simulink model "qr_array"  (R2017a)
settings: Solver=VariableStepAuto  StartTime=0.0  StopTime=777  RelTol=1e-3
libraries: xbsIndex_r4 x646
(part 2 of 4)

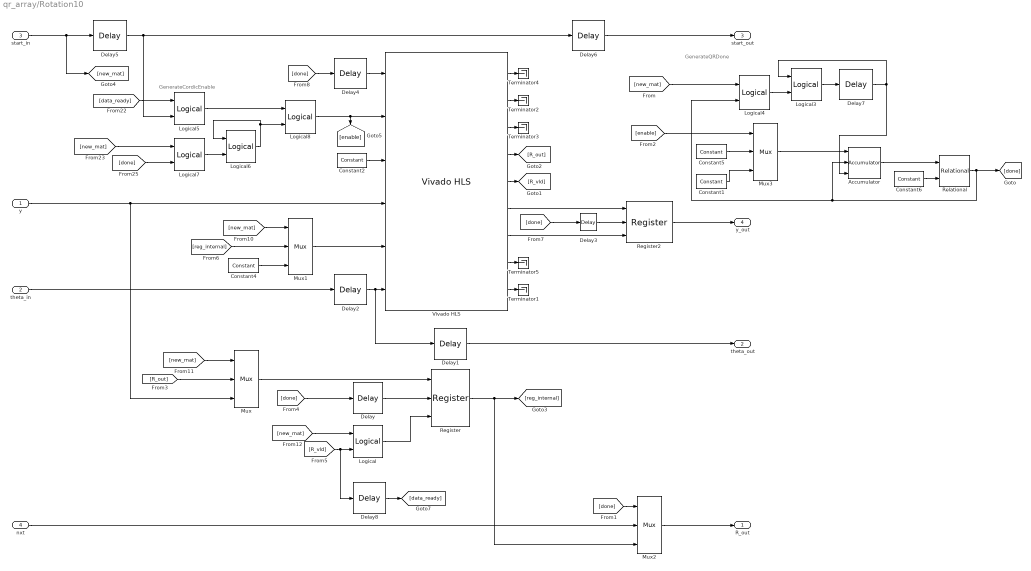
== system qr_array/Rotation10 ==
  note: GenerateQRDone
  note: GenerateCordicEnable
  y : Inport
  theta_in : Inport  Port=2
  start_in : Inport  Port=3
  nxt : Inport  Port=4
  Accumulator : xbsIndex_r4/Accumulator  operation=Add  n_bits=8  overflow=Wrap  scale=1  rst=on  hasbypass=off  infoeditControl=reset for floating point data type must be asserted for a minimum of 2 cycles  en=on  latency=1  msb_inp=100  msb=100  lsb=-100  use_behavioral_HDL=on  implementation=Fabric  dbl_ovrd=off  block_type=accum
  Constant1 : xbsIndex_r4/Constant  const=1  gui_display_data_type=Fixed-point  arith_type=Unsigned  n_bits=16  bin_pt=0  preci_type=Single  exp_width=8  frac_width=24  explicit_period=off  period=1  equ=P=C  opselect=C  inp2=PCIN>>17  opr=+  inp1=P  carry=CIN  dbl_ovrd=off  block_type=constant
  Constant2 : xbsIndex_r4/Constant  const=1  gui_display_data_type=Boolean  arith_type=Boolean  n_bits=16  bin_pt=14  preci_type=Single  exp_width=8  frac_width=24  explicit_period=off  period=1  equ=P=C  opselect=C  inp2=PCIN>>17  opr=+  inp1=P  carry=CIN  dbl_ovrd=off  block_type=constant
  Constant4 : xbsIndex_r4/Constant  const=0  gui_display_data_type=Fixed-point  arith_type=Signed (2's comp)  n_bits=16  bin_pt=13  preci_type=Single  exp_width=8  frac_width=24  explicit_period=off  period=1  equ=P=C  opselect=C  inp2=PCIN>>17  opr=+  inp1=P  carry=CIN  dbl_ovrd=off  block_type=constant
  Constant5 : xbsIndex_r4/Constant  const=0  gui_display_data_type=Fixed-point  arith_type=Unsigned  n_bits=16  bin_pt=0  preci_type=Single  exp_width=8  frac_width=24  explicit_period=off  period=1  equ=P=C  opselect=C  inp2=PCIN>>17  opr=+  inp1=P  carry=CIN  dbl_ovrd=off  block_type=constant
  Constant6 : xbsIndex_r4/Constant  const=3  gui_display_data_type=Fixed-point  arith_type=Unsigned  n_bits=16  bin_pt=0  preci_type=Single  exp_width=8  frac_width=24  explicit_period=off  period=1  equ=P=C  opselect=C  inp2=PCIN>>17  opr=+  inp1=P  carry=CIN  dbl_ovrd=off  block_type=constant
  Delay{,3,6..7} (4 alike) : xbsIndex_r4/Delay  rst=off  infoeditControl=Selection of Reset will increase slice count due to use of real FFs and instead of SRLs  en=off  latency=1  reg_retiming=off  dbl_ovrd=off  block_type=delay
  Delay1 : xbsIndex_r4/Delay  rst=off  infoeditControl=Selection of Reset will increase slice count due to use of real FFs and instead of SRLs  en=off  latency=41  reg_retiming=off  dbl_ovrd=off  block_type=delay
  Delay2 : xbsIndex_r4/Delay  rst=off  infoeditControl=Selection of Reset will increase slice count due to use of real FFs and instead of SRLs  en=off  latency=2  reg_retiming=off  dbl_ovrd=off  block_type=delay
  Delay4 : xbsIndex_r4/Delay  rst=off  infoeditControl=Selection of Reset will increase slice count due to use of real FFs and instead of SRLs  en=off  latency=4  reg_retiming=off  dbl_ovrd=off  block_type=delay
  Delay5 : xbsIndex_r4/Delay  rst=off  infoeditControl=Selection of Reset will increase slice count due to use of real FFs and instead of SRLs  en=off  latency=43  reg_retiming=off  dbl_ovrd=off  block_type=delay
  Delay8 : xbsIndex_r4/Delay  rst=off  infoeditControl=Selection of Reset will increase slice count due to use of real FFs and instead of SRLs  en=off  latency=2  reg_retiming=off  dbl_ovrd=off  block_type=delay
  Logical : xbsIndex_r4/Logical  logical_function=OR  inputs=2  en=off  latency=1  precision=Full  arith_type=Unsigned  n_bits=16  bin_pt=0  align_bp=on  dbl_ovrd=off  block_type=logical
  Logical3 : xbsIndex_r4/Logical  logical_function=XOR  inputs=2  en=off  latency=0  precision=Full  arith_type=Unsigned  n_bits=16  bin_pt=0  align_bp=on  dbl_ovrd=off  block_type=logical
  Logical4 : xbsIndex_r4/Logical  logical_function=OR  inputs=2  en=off  latency=1  precision=Full  arith_type=Unsigned  n_bits=16  bin_pt=0  align_bp=on  dbl_ovrd=off  block_type=logical
  Logical5 : xbsIndex_r4/Logical  logical_function=OR  inputs=2  en=off  latency=0  precision=Full  arith_type=Unsigned  n_bits=16  bin_pt=0  align_bp=on  dbl_ovrd=off  block_type=logical
  Logical6 : xbsIndex_r4/Logical  logical_function=XOR  inputs=2  en=off  latency=1  precision=Full  arith_type=Unsigned  n_bits=16  bin_pt=0  align_bp=on  dbl_ovrd=off  block_type=logical
  Logical7 : xbsIndex_r4/Logical  logical_function=OR  inputs=2  en=off  latency=1  precision=Full  arith_type=Unsigned  n_bits=16  bin_pt=0  align_bp=on  dbl_ovrd=off  block_type=logical
  Logical8 : xbsIndex_r4/Logical  logical_function=AND  inputs=2  en=off  latency=1  precision=Full  arith_type=Unsigned  n_bits=16  bin_pt=0  align_bp=on  dbl_ovrd=off  block_type=logical
  Mux{,1..3} (4 alike) : xbsIndex_r4/Mux  inputs=2  en=off  latency=1  precision=Full  arith_type=Unsigned  n_bits=16  bin_pt=14  quantization=Truncate  overflow=Wrap  dbl_ovrd=off  block_type=mux
  Register : xbsIndex_r4/Register  init=0  rst=on  en=on  dbl_ovrd=off  block_type=register
  Register2 : xbsIndex_r4/Register  init=0  rst=on  en=on  dbl_ovrd=off  block_type=register
  Relational : xbsIndex_r4/Relational  mode=a=b  op_type=Bool  en=off  latency=0  dbl_ovrd=off  block_type=relational
  Terminator{1..5} (5 alike) : Terminator
  Vivado HLS : xbsIndex_r4/Vivado HLS  anytable='C:/ELEC522/hellar/Project_4/cordic_revised/cordic_revised/solution1'  fast_sim=off  display_datatype=on  rate_propagation_method=Simulink system period  model_file_path=''  latency=1  block_type=hls
      settings: infoedit=This block allows including C,C++ and SystemC source files in System Generator for DSP designs.
  R_out : Outport
  theta_out : Outport  Port=2
  start_out : Outport  Port=3
  y_out : Outport  Port=4
  wires:
  [done] -> Delay3/1
  Delay8/1 -> [data_ready]
  [R_vld] -> Delay8/1, Logical/2
  [done] -> Mux2/1
  [new_mat] -> Mux/1
  [done] -> Delay4/1
  [new_mat] -> Mux1/1
  [reg_internal] -> Mux1/2
  Delay4/1 -> Vivado HLS/1
  Logical/1 -> Register/3
  [done] -> Delay/1
  [new_mat] -> Logical/1
  theta_in/1 -> Delay2/1
  Register/1 -> Mux2/3, [reg_internal]
  Delay6/1 -> start_out/1
  Mux/1 -> Register/1
  Vivado HLS/3 -> Terminator3/1
  Vivado HLS/5 -> [R_vld]
  [R_out] -> Mux/2
  Delay/1 -> Register/2
  y/1 -> Vivado HLS/4, Mux/3
  Vivado HLS/1 -> Terminator4/1
  Vivado HLS/4 -> [R_out]
  Mux2/1 -> R_out/1
  Constant4/1 -> Mux1/3
  start_in/1 -> [new_mat], Delay5/1
  nxt/1 -> Mux2/2
  Vivado HLS/2 -> Terminator2/1
  Constant2/1 -> Vivado HLS/3
  Logical8/1 -> Vivado HLS/2, [enable]
  Relational/1 -> Logical4/2, Accumulator/2, [done]
  Vivado HLS/8 -> Terminator5/1
  Vivado HLS/9 -> Terminator1/1
  Vivado HLS/6 -> Register2/1
  Vivado HLS/7 -> Register2/3
  Delay1/1 -> theta_out/1
  Delay2/1 -> Delay1/1, Vivado HLS/6
  Mux1/1 -> Vivado HLS/5
  Delay3/1 -> Register2/2
  Register2/1 -> y_out/1
  Logical5/1 -> Logical8/1
  Logical7/1 -> Logical6/2
  Logical6/1 -> Logical6/1, Logical8/2
  [done] -> Logical7/2
  [new_mat] -> Logical7/1
  [data_ready] -> Logical5/1
  Delay5/1 -> Delay6/1, Logical5/2
  Delay7/1 -> Logical3/1, Accumulator/3
  Logical3/1 -> Delay7/1
  Logical4/1 -> Logical3/2
  [new_mat] -> Logical4/1
  Constant6/1 -> Relational/2
  Constant5/1 -> Mux3/2
  Constant1/1 -> Mux3/3
  Accumulator/1 -> Relational/1
  Mux3/1 -> Accumulator/1
  [enable] -> Mux3/1

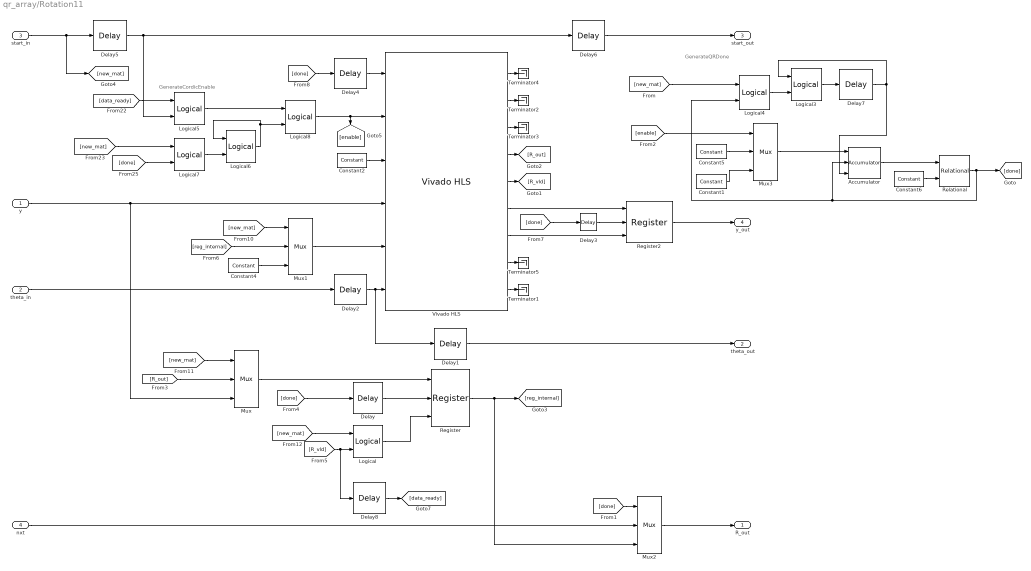
== system qr_array/Rotation11 ==
  note: GenerateQRDone
  note: GenerateCordicEnable
  y : Inport
  theta_in : Inport  Port=2
  start_in : Inport  Port=3
  nxt : Inport  Port=4
  Accumulator : xbsIndex_r4/Accumulator  operation=Add  n_bits=8  overflow=Wrap  scale=1  rst=on  hasbypass=off  infoeditControl=reset for floating point data type must be asserted for a minimum of 2 cycles  en=on  latency=1  msb_inp=100  msb=100  lsb=-100  use_behavioral_HDL=on  implementation=Fabric  dbl_ovrd=off  block_type=accum
  Constant1 : xbsIndex_r4/Constant  const=1  gui_display_data_type=Fixed-point  arith_type=Unsigned  n_bits=16  bin_pt=0  preci_type=Single  exp_width=8  frac_width=24  explicit_period=off  period=1  equ=P=C  opselect=C  inp2=PCIN>>17  opr=+  inp1=P  carry=CIN  dbl_ovrd=off  block_type=constant
  Constant2 : xbsIndex_r4/Constant  const=1  gui_display_data_type=Boolean  arith_type=Boolean  n_bits=16  bin_pt=14  preci_type=Single  exp_width=8  frac_width=24  explicit_period=off  period=1  equ=P=C  opselect=C  inp2=PCIN>>17  opr=+  inp1=P  carry=CIN  dbl_ovrd=off  block_type=constant
  Constant4 : xbsIndex_r4/Constant  const=0  gui_display_data_type=Fixed-point  arith_type=Signed (2's comp)  n_bits=16  bin_pt=13  preci_type=Single  exp_width=8  frac_width=24  explicit_period=off  period=1  equ=P=C  opselect=C  inp2=PCIN>>17  opr=+  inp1=P  carry=CIN  dbl_ovrd=off  block_type=constant
  Constant5 : xbsIndex_r4/Constant  const=0  gui_display_data_type=Fixed-point  arith_type=Unsigned  n_bits=16  bin_pt=0  preci_type=Single  exp_width=8  frac_width=24  explicit_period=off  period=1  equ=P=C  opselect=C  inp2=PCIN>>17  opr=+  inp1=P  carry=CIN  dbl_ovrd=off  block_type=constant
  Constant6 : xbsIndex_r4/Constant  const=3  gui_display_data_type=Fixed-point  arith_type=Unsigned  n_bits=16  bin_pt=0  preci_type=Single  exp_width=8  frac_width=24  explicit_period=off  period=1  equ=P=C  opselect=C  inp2=PCIN>>17  opr=+  inp1=P  carry=CIN  dbl_ovrd=off  block_type=constant
  Delay{,3,6..7} (4 alike) : xbsIndex_r4/Delay  rst=off  infoeditControl=Selection of Reset will increase slice count due to use of real FFs and instead of SRLs  en=off  latency=1  reg_retiming=off  dbl_ovrd=off  block_type=delay
  Delay1 : xbsIndex_r4/Delay  rst=off  infoeditControl=Selection of Reset will increase slice count due to use of real FFs and instead of SRLs  en=off  latency=41  reg_retiming=off  dbl_ovrd=off  block_type=delay
  Delay2 : xbsIndex_r4/Delay  rst=off  infoeditControl=Selection of Reset will increase slice count due to use of real FFs and instead of SRLs  en=off  latency=2  reg_retiming=off  dbl_ovrd=off  block_type=delay
  Delay4 : xbsIndex_r4/Delay  rst=off  infoeditControl=Selection of Reset will increase slice count due to use of real FFs and instead of SRLs  en=off  latency=4  reg_retiming=off  dbl_ovrd=off  block_type=delay
  Delay5 : xbsIndex_r4/Delay  rst=off  infoeditControl=Selection of Reset will increase slice count due to use of real FFs and instead of SRLs  en=off  latency=43  reg_retiming=off  dbl_ovrd=off  block_type=delay
  Delay8 : xbsIndex_r4/Delay  rst=off  infoeditControl=Selection of Reset will increase slice count due to use of real FFs and instead of SRLs  en=off  latency=2  reg_retiming=off  dbl_ovrd=off  block_type=delay
  Logical : xbsIndex_r4/Logical  logical_function=OR  inputs=2  en=off  latency=1  precision=Full  arith_type=Unsigned  n_bits=16  bin_pt=0  align_bp=on  dbl_ovrd=off  block_type=logical
  Logical3 : xbsIndex_r4/Logical  logical_function=XOR  inputs=2  en=off  latency=0  precision=Full  arith_type=Unsigned  n_bits=16  bin_pt=0  align_bp=on  dbl_ovrd=off  block_type=logical
  Logical4 : xbsIndex_r4/Logical  logical_function=OR  inputs=2  en=off  latency=1  precision=Full  arith_type=Unsigned  n_bits=16  bin_pt=0  align_bp=on  dbl_ovrd=off  block_type=logical
  Logical5 : xbsIndex_r4/Logical  logical_function=OR  inputs=2  en=off  latency=0  precision=Full  arith_type=Unsigned  n_bits=16  bin_pt=0  align_bp=on  dbl_ovrd=off  block_type=logical
  Logical6 : xbsIndex_r4/Logical  logical_function=XOR  inputs=2  en=off  latency=1  precision=Full  arith_type=Unsigned  n_bits=16  bin_pt=0  align_bp=on  dbl_ovrd=off  block_type=logical
  Logical7 : xbsIndex_r4/Logical  logical_function=OR  inputs=2  en=off  latency=1  precision=Full  arith_type=Unsigned  n_bits=16  bin_pt=0  align_bp=on  dbl_ovrd=off  block_type=logical
  Logical8 : xbsIndex_r4/Logical  logical_function=AND  inputs=2  en=off  latency=1  precision=Full  arith_type=Unsigned  n_bits=16  bin_pt=0  align_bp=on  dbl_ovrd=off  block_type=logical
  Mux{,1..3} (4 alike) : xbsIndex_r4/Mux  inputs=2  en=off  latency=1  precision=Full  arith_type=Unsigned  n_bits=16  bin_pt=14  quantization=Truncate  overflow=Wrap  dbl_ovrd=off  block_type=mux
  Register : xbsIndex_r4/Register  init=0  rst=on  en=on  dbl_ovrd=off  block_type=register
  Register2 : xbsIndex_r4/Register  init=0  rst=on  en=on  dbl_ovrd=off  block_type=register
  Relational : xbsIndex_r4/Relational  mode=a=b  op_type=Bool  en=off  latency=0  dbl_ovrd=off  block_type=relational
  Terminator{1..5} (5 alike) : Terminator
  Vivado HLS : xbsIndex_r4/Vivado HLS  anytable='C:/ELEC522/hellar/Project_4/cordic_revised/cordic_revised/solution1'  fast_sim=off  display_datatype=on  rate_propagation_method=Simulink system period  model_file_path=''  latency=1  block_type=hls
      settings: infoedit=This block allows including C,C++ and SystemC source files in System Generator for DSP designs.
  R_out : Outport
  theta_out : Outport  Port=2
  start_out : Outport  Port=3
  y_out : Outport  Port=4
  wires:
  [done] -> Delay3/1
  Delay8/1 -> [data_ready]
  [R_vld] -> Delay8/1, Logical/2
  [done] -> Mux2/1
  [new_mat] -> Mux/1
  [done] -> Delay4/1
  [new_mat] -> Mux1/1
  [reg_internal] -> Mux1/2
  Delay4/1 -> Vivado HLS/1
  Logical/1 -> Register/3
  [done] -> Delay/1
  [new_mat] -> Logical/1
  theta_in/1 -> Delay2/1
  Register/1 -> Mux2/3, [reg_internal]
  Delay6/1 -> start_out/1
  Mux/1 -> Register/1
  Vivado HLS/3 -> Terminator3/1
  Vivado HLS/5 -> [R_vld]
  [R_out] -> Mux/2
  Delay/1 -> Register/2
  y/1 -> Vivado HLS/4, Mux/3
  Vivado HLS/1 -> Terminator4/1
  Vivado HLS/4 -> [R_out]
  Mux2/1 -> R_out/1
  Constant4/1 -> Mux1/3
  start_in/1 -> [new_mat], Delay5/1
  nxt/1 -> Mux2/2
  Vivado HLS/2 -> Terminator2/1
  Constant2/1 -> Vivado HLS/3
  Logical8/1 -> Vivado HLS/2, [enable]
  Relational/1 -> Logical4/2, Accumulator/2, [done]
  Vivado HLS/8 -> Terminator5/1
  Vivado HLS/9 -> Terminator1/1
  Vivado HLS/6 -> Register2/1
  Vivado HLS/7 -> Register2/3
  Delay1/1 -> theta_out/1
  Delay2/1 -> Delay1/1, Vivado HLS/6
  Mux1/1 -> Vivado HLS/5
  Delay3/1 -> Register2/2
  Register2/1 -> y_out/1
  Logical5/1 -> Logical8/1
  Logical7/1 -> Logical6/2
  Logical6/1 -> Logical6/1, Logical8/2
  [done] -> Logical7/2
  [new_mat] -> Logical7/1
  [data_ready] -> Logical5/1
  Delay5/1 -> Delay6/1, Logical5/2
  Delay7/1 -> Logical3/1, Accumulator/3
  Logical3/1 -> Delay7/1
  Logical4/1 -> Logical3/2
  [new_mat] -> Logical4/1
  Constant6/1 -> Relational/2
  Constant5/1 -> Mux3/2
  Constant1/1 -> Mux3/3
  Accumulator/1 -> Relational/1
  Mux3/1 -> Accumulator/1
  [enable] -> Mux3/1

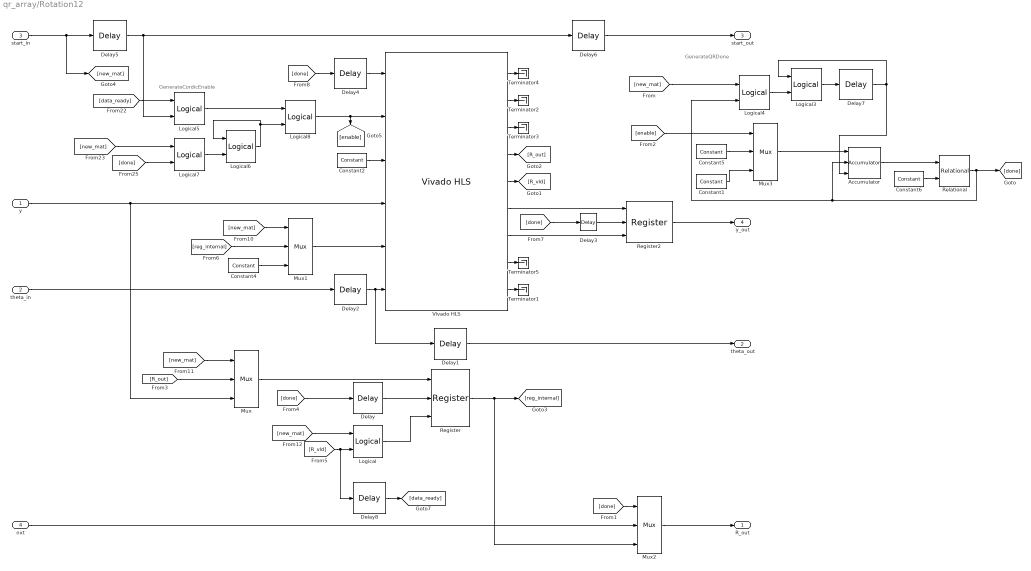
== system qr_array/Rotation12 ==
  note: GenerateQRDone
  note: GenerateCordicEnable
  y : Inport
  theta_in : Inport  Port=2
  start_in : Inport  Port=3
  nxt : Inport  Port=4
  Accumulator : xbsIndex_r4/Accumulator  operation=Add  n_bits=8  overflow=Wrap  scale=1  rst=on  hasbypass=off  infoeditControl=reset for floating point data type must be asserted for a minimum of 2 cycles  en=on  latency=1  msb_inp=100  msb=100  lsb=-100  use_behavioral_HDL=on  implementation=Fabric  dbl_ovrd=off  block_type=accum
  Constant1 : xbsIndex_r4/Constant  const=1  gui_display_data_type=Fixed-point  arith_type=Unsigned  n_bits=16  bin_pt=0  preci_type=Single  exp_width=8  frac_width=24  explicit_period=off  period=1  equ=P=C  opselect=C  inp2=PCIN>>17  opr=+  inp1=P  carry=CIN  dbl_ovrd=off  block_type=constant
  Constant2 : xbsIndex_r4/Constant  const=1  gui_display_data_type=Boolean  arith_type=Boolean  n_bits=16  bin_pt=14  preci_type=Single  exp_width=8  frac_width=24  explicit_period=off  period=1  equ=P=C  opselect=C  inp2=PCIN>>17  opr=+  inp1=P  carry=CIN  dbl_ovrd=off  block_type=constant
  Constant4 : xbsIndex_r4/Constant  const=0  gui_display_data_type=Fixed-point  arith_type=Signed (2's comp)  n_bits=16  bin_pt=13  preci_type=Single  exp_width=8  frac_width=24  explicit_period=off  period=1  equ=P=C  opselect=C  inp2=PCIN>>17  opr=+  inp1=P  carry=CIN  dbl_ovrd=off  block_type=constant
  Constant5 : xbsIndex_r4/Constant  const=0  gui_display_data_type=Fixed-point  arith_type=Unsigned  n_bits=16  bin_pt=0  preci_type=Single  exp_width=8  frac_width=24  explicit_period=off  period=1  equ=P=C  opselect=C  inp2=PCIN>>17  opr=+  inp1=P  carry=CIN  dbl_ovrd=off  block_type=constant
  Constant6 : xbsIndex_r4/Constant  const=2  gui_display_data_type=Fixed-point  arith_type=Unsigned  n_bits=16  bin_pt=0  preci_type=Single  exp_width=8  frac_width=24  explicit_period=off  period=1  equ=P=C  opselect=C  inp2=PCIN>>17  opr=+  inp1=P  carry=CIN  dbl_ovrd=off  block_type=constant
  Delay{,3,6..7} (4 alike) : xbsIndex_r4/Delay  rst=off  infoeditControl=Selection of Reset will increase slice count due to use of real FFs and instead of SRLs  en=off  latency=1  reg_retiming=off  dbl_ovrd=off  block_type=delay
  Delay1 : xbsIndex_r4/Delay  rst=off  infoeditControl=Selection of Reset will increase slice count due to use of real FFs and instead of SRLs  en=off  latency=41  reg_retiming=off  dbl_ovrd=off  block_type=delay
  Delay2 : xbsIndex_r4/Delay  rst=off  infoeditControl=Selection of Reset will increase slice count due to use of real FFs and instead of SRLs  en=off  latency=2  reg_retiming=off  dbl_ovrd=off  block_type=delay
  Delay4 : xbsIndex_r4/Delay  rst=off  infoeditControl=Selection of Reset will increase slice count due to use of real FFs and instead of SRLs  en=off  latency=4  reg_retiming=off  dbl_ovrd=off  block_type=delay
  Delay5 : xbsIndex_r4/Delay  rst=off  infoeditControl=Selection of Reset will increase slice count due to use of real FFs and instead of SRLs  en=off  latency=43  reg_retiming=off  dbl_ovrd=off  block_type=delay
  Delay8 : xbsIndex_r4/Delay  rst=off  infoeditControl=Selection of Reset will increase slice count due to use of real FFs and instead of SRLs  en=off  latency=2  reg_retiming=off  dbl_ovrd=off  block_type=delay
  Logical : xbsIndex_r4/Logical  logical_function=OR  inputs=2  en=off  latency=1  precision=Full  arith_type=Unsigned  n_bits=16  bin_pt=0  align_bp=on  dbl_ovrd=off  block_type=logical
  Logical3 : xbsIndex_r4/Logical  logical_function=XOR  inputs=2  en=off  latency=0  precision=Full  arith_type=Unsigned  n_bits=16  bin_pt=0  align_bp=on  dbl_ovrd=off  block_type=logical
  Logical4 : xbsIndex_r4/Logical  logical_function=OR  inputs=2  en=off  latency=1  precision=Full  arith_type=Unsigned  n_bits=16  bin_pt=0  align_bp=on  dbl_ovrd=off  block_type=logical
  Logical5 : xbsIndex_r4/Logical  logical_function=OR  inputs=2  en=off  latency=0  precision=Full  arith_type=Unsigned  n_bits=16  bin_pt=0  align_bp=on  dbl_ovrd=off  block_type=logical
  Logical6 : xbsIndex_r4/Logical  logical_function=XOR  inputs=2  en=off  latency=1  precision=Full  arith_type=Unsigned  n_bits=16  bin_pt=0  align_bp=on  dbl_ovrd=off  block_type=logical
  Logical7 : xbsIndex_r4/Logical  logical_function=OR  inputs=2  en=off  latency=1  precision=Full  arith_type=Unsigned  n_bits=16  bin_pt=0  align_bp=on  dbl_ovrd=off  block_type=logical
  Logical8 : xbsIndex_r4/Logical  logical_function=AND  inputs=2  en=off  latency=1  precision=Full  arith_type=Unsigned  n_bits=16  bin_pt=0  align_bp=on  dbl_ovrd=off  block_type=logical
  Mux{,1..3} (4 alike) : xbsIndex_r4/Mux  inputs=2  en=off  latency=1  precision=Full  arith_type=Unsigned  n_bits=16  bin_pt=14  quantization=Truncate  overflow=Wrap  dbl_ovrd=off  block_type=mux
  Register : xbsIndex_r4/Register  init=0  rst=on  en=on  dbl_ovrd=off  block_type=register
  Register2 : xbsIndex_r4/Register  init=0  rst=on  en=on  dbl_ovrd=off  block_type=register
  Relational : xbsIndex_r4/Relational  mode=a=b  op_type=Bool  en=off  latency=0  dbl_ovrd=off  block_type=relational
  Terminator{1..5} (5 alike) : Terminator
  Vivado HLS : xbsIndex_r4/Vivado HLS  anytable='C:/ELEC522/hellar/Project_4/cordic_revised/cordic_revised/solution1'  fast_sim=off  display_datatype=on  rate_propagation_method=Simulink system period  model_file_path=''  latency=1  block_type=hls
      settings: infoedit=This block allows including C,C++ and SystemC source files in System Generator for DSP designs.
  R_out : Outport
  theta_out : Outport  Port=2
  start_out : Outport  Port=3
  y_out : Outport  Port=4
  wires:
  [done] -> Delay3/1
  Delay8/1 -> [data_ready]
  [R_vld] -> Delay8/1, Logical/2
  [done] -> Mux2/1
  [new_mat] -> Mux/1
  [done] -> Delay4/1
  [new_mat] -> Mux1/1
  [reg_internal] -> Mux1/2
  Delay4/1 -> Vivado HLS/1
  Logical/1 -> Register/3
  [done] -> Delay/1
  [new_mat] -> Logical/1
  theta_in/1 -> Delay2/1
  Register/1 -> Mux2/3, [reg_internal]
  Delay6/1 -> start_out/1
  Mux/1 -> Register/1
  Vivado HLS/3 -> Terminator3/1
  Vivado HLS/5 -> [R_vld]
  [R_out] -> Mux/2
  Delay/1 -> Register/2
  y/1 -> Vivado HLS/4, Mux/3
  Vivado HLS/1 -> Terminator4/1
  Vivado HLS/4 -> [R_out]
  Mux2/1 -> R_out/1
  Constant4/1 -> Mux1/3
  start_in/1 -> [new_mat], Delay5/1
  nxt/1 -> Mux2/2
  Vivado HLS/2 -> Terminator2/1
  Constant2/1 -> Vivado HLS/3
  Logical8/1 -> Vivado HLS/2, [enable]
  Relational/1 -> Logical4/2, Accumulator/2, [done]
  Vivado HLS/8 -> Terminator5/1
  Vivado HLS/9 -> Terminator1/1
  Vivado HLS/6 -> Register2/1
  Vivado HLS/7 -> Register2/3
  Delay1/1 -> theta_out/1
  Delay2/1 -> Delay1/1, Vivado HLS/6
  Mux1/1 -> Vivado HLS/5
  Delay3/1 -> Register2/2
  Register2/1 -> y_out/1
  Logical5/1 -> Logical8/1
  Logical7/1 -> Logical6/2
  Logical6/1 -> Logical6/1, Logical8/2
  [done] -> Logical7/2
  [new_mat] -> Logical7/1
  [data_ready] -> Logical5/1
  Delay5/1 -> Delay6/1, Logical5/2
  Delay7/1 -> Logical3/1, Accumulator/3
  Logical3/1 -> Delay7/1
  Logical4/1 -> Logical3/2
  [new_mat] -> Logical4/1
  Constant6/1 -> Relational/2
  Constant5/1 -> Mux3/2
  Constant1/1 -> Mux3/3
  Accumulator/1 -> Relational/1
  Mux3/1 -> Accumulator/1
  [enable] -> Mux3/1

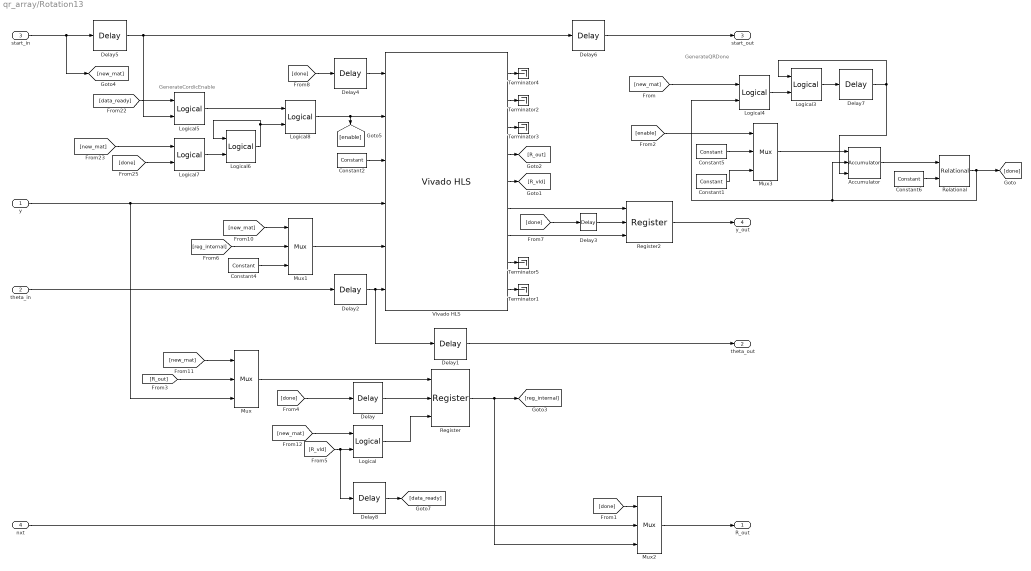
== system qr_array/Rotation13 ==
  note: GenerateQRDone
  note: GenerateCordicEnable
  y : Inport
  theta_in : Inport  Port=2
  start_in : Inport  Port=3
  nxt : Inport  Port=4
  Accumulator : xbsIndex_r4/Accumulator  operation=Add  n_bits=8  overflow=Wrap  scale=1  rst=on  hasbypass=off  infoeditControl=reset for floating point data type must be asserted for a minimum of 2 cycles  en=on  latency=1  msb_inp=100  msb=100  lsb=-100  use_behavioral_HDL=on  implementation=Fabric  dbl_ovrd=off  block_type=accum
  Constant1 : xbsIndex_r4/Constant  const=1  gui_display_data_type=Fixed-point  arith_type=Unsigned  n_bits=16  bin_pt=0  preci_type=Single  exp_width=8  frac_width=24  explicit_period=off  period=1  equ=P=C  opselect=C  inp2=PCIN>>17  opr=+  inp1=P  carry=CIN  dbl_ovrd=off  block_type=constant
  Constant2 : xbsIndex_r4/Constant  const=1  gui_display_data_type=Boolean  arith_type=Boolean  n_bits=16  bin_pt=14  preci_type=Single  exp_width=8  frac_width=24  explicit_period=off  period=1  equ=P=C  opselect=C  inp2=PCIN>>17  opr=+  inp1=P  carry=CIN  dbl_ovrd=off  block_type=constant
  Constant4 : xbsIndex_r4/Constant  const=0  gui_display_data_type=Fixed-point  arith_type=Signed (2's comp)  n_bits=16  bin_pt=13  preci_type=Single  exp_width=8  frac_width=24  explicit_period=off  period=1  equ=P=C  opselect=C  inp2=PCIN>>17  opr=+  inp1=P  carry=CIN  dbl_ovrd=off  block_type=constant
  Constant5 : xbsIndex_r4/Constant  const=0  gui_display_data_type=Fixed-point  arith_type=Unsigned  n_bits=16  bin_pt=0  preci_type=Single  exp_width=8  frac_width=24  explicit_period=off  period=1  equ=P=C  opselect=C  inp2=PCIN>>17  opr=+  inp1=P  carry=CIN  dbl_ovrd=off  block_type=constant
  Constant6 : xbsIndex_r4/Constant  const=2  gui_display_data_type=Fixed-point  arith_type=Unsigned  n_bits=16  bin_pt=0  preci_type=Single  exp_width=8  frac_width=24  explicit_period=off  period=1  equ=P=C  opselect=C  inp2=PCIN>>17  opr=+  inp1=P  carry=CIN  dbl_ovrd=off  block_type=constant
  Delay{,3,6..7} (4 alike) : xbsIndex_r4/Delay  rst=off  infoeditControl=Selection of Reset will increase slice count due to use of real FFs and instead of SRLs  en=off  latency=1  reg_retiming=off  dbl_ovrd=off  block_type=delay
  Delay1 : xbsIndex_r4/Delay  rst=off  infoeditControl=Selection of Reset will increase slice count due to use of real FFs and instead of SRLs  en=off  latency=41  reg_retiming=off  dbl_ovrd=off  block_type=delay
  Delay2 : xbsIndex_r4/Delay  rst=off  infoeditControl=Selection of Reset will increase slice count due to use of real FFs and instead of SRLs  en=off  latency=2  reg_retiming=off  dbl_ovrd=off  block_type=delay
  Delay4 : xbsIndex_r4/Delay  rst=off  infoeditControl=Selection of Reset will increase slice count due to use of real FFs and instead of SRLs  en=off  latency=4  reg_retiming=off  dbl_ovrd=off  block_type=delay
  Delay5 : xbsIndex_r4/Delay  rst=off  infoeditControl=Selection of Reset will increase slice count due to use of real FFs and instead of SRLs  en=off  latency=43  reg_retiming=off  dbl_ovrd=off  block_type=delay
  Delay8 : xbsIndex_r4/Delay  rst=off  infoeditControl=Selection of Reset will increase slice count due to use of real FFs and instead of SRLs  en=off  latency=2  reg_retiming=off  dbl_ovrd=off  block_type=delay
  Logical : xbsIndex_r4/Logical  logical_function=OR  inputs=2  en=off  latency=1  precision=Full  arith_type=Unsigned  n_bits=16  bin_pt=0  align_bp=on  dbl_ovrd=off  block_type=logical
  Logical3 : xbsIndex_r4/Logical  logical_function=XOR  inputs=2  en=off  latency=0  precision=Full  arith_type=Unsigned  n_bits=16  bin_pt=0  align_bp=on  dbl_ovrd=off  block_type=logical
  Logical4 : xbsIndex_r4/Logical  logical_function=OR  inputs=2  en=off  latency=1  precision=Full  arith_type=Unsigned  n_bits=16  bin_pt=0  align_bp=on  dbl_ovrd=off  block_type=logical
  Logical5 : xbsIndex_r4/Logical  logical_function=OR  inputs=2  en=off  latency=0  precision=Full  arith_type=Unsigned  n_bits=16  bin_pt=0  align_bp=on  dbl_ovrd=off  block_type=logical
  Logical6 : xbsIndex_r4/Logical  logical_function=XOR  inputs=2  en=off  latency=1  precision=Full  arith_type=Unsigned  n_bits=16  bin_pt=0  align_bp=on  dbl_ovrd=off  block_type=logical
  Logical7 : xbsIndex_r4/Logical  logical_function=OR  inputs=2  en=off  latency=1  precision=Full  arith_type=Unsigned  n_bits=16  bin_pt=0  align_bp=on  dbl_ovrd=off  block_type=logical
  Logical8 : xbsIndex_r4/Logical  logical_function=AND  inputs=2  en=off  latency=1  precision=Full  arith_type=Unsigned  n_bits=16  bin_pt=0  align_bp=on  dbl_ovrd=off  block_type=logical
  Mux{,1..3} (4 alike) : xbsIndex_r4/Mux  inputs=2  en=off  latency=1  precision=Full  arith_type=Unsigned  n_bits=16  bin_pt=14  quantization=Truncate  overflow=Wrap  dbl_ovrd=off  block_type=mux
  Register : xbsIndex_r4/Register  init=0  rst=on  en=on  dbl_ovrd=off  block_type=register
  Register2 : xbsIndex_r4/Register  init=0  rst=on  en=on  dbl_ovrd=off  block_type=register
  Relational : xbsIndex_r4/Relational  mode=a=b  op_type=Bool  en=off  latency=0  dbl_ovrd=off  block_type=relational
  Terminator{1..5} (5 alike) : Terminator
  Vivado HLS : xbsIndex_r4/Vivado HLS  anytable='C:/ELEC522/hellar/Project_4/cordic_revised/cordic_revised/solution1'  fast_sim=off  display_datatype=on  rate_propagation_method=Simulink system period  model_file_path=''  latency=1  block_type=hls
      settings: infoedit=This block allows including C,C++ and SystemC source files in System Generator for DSP designs.
  R_out : Outport
  theta_out : Outport  Port=2
  start_out : Outport  Port=3
  y_out : Outport  Port=4
  wires:
  [done] -> Delay3/1
  Delay8/1 -> [data_ready]
  [R_vld] -> Delay8/1, Logical/2
  [done] -> Mux2/1
  [new_mat] -> Mux/1
  [done] -> Delay4/1
  [new_mat] -> Mux1/1
  [reg_internal] -> Mux1/2
  Delay4/1 -> Vivado HLS/1
  Logical/1 -> Register/3
  [done] -> Delay/1
  [new_mat] -> Logical/1
  theta_in/1 -> Delay2/1
  Register/1 -> Mux2/3, [reg_internal]
  Delay6/1 -> start_out/1
  Mux/1 -> Register/1
  Vivado HLS/3 -> Terminator3/1
  Vivado HLS/5 -> [R_vld]
  [R_out] -> Mux/2
  Delay/1 -> Register/2
  y/1 -> Vivado HLS/4, Mux/3
  Vivado HLS/1 -> Terminator4/1
  Vivado HLS/4 -> [R_out]
  Mux2/1 -> R_out/1
  Constant4/1 -> Mux1/3
  start_in/1 -> [new_mat], Delay5/1
  nxt/1 -> Mux2/2
  Vivado HLS/2 -> Terminator2/1
  Constant2/1 -> Vivado HLS/3
  Logical8/1 -> Vivado HLS/2, [enable]
  Relational/1 -> Logical4/2, Accumulator/2, [done]
  Vivado HLS/8 -> Terminator5/1
  Vivado HLS/9 -> Terminator1/1
  Vivado HLS/6 -> Register2/1
  Vivado HLS/7 -> Register2/3
  Delay1/1 -> theta_out/1
  Delay2/1 -> Delay1/1, Vivado HLS/6
  Mux1/1 -> Vivado HLS/5
  Delay3/1 -> Register2/2
  Register2/1 -> y_out/1
  Logical5/1 -> Logical8/1
  Logical7/1 -> Logical6/2
  Logical6/1 -> Logical6/1, Logical8/2
  [done] -> Logical7/2
  [new_mat] -> Logical7/1
  [data_ready] -> Logical5/1
  Delay5/1 -> Delay6/1, Logical5/2
  Delay7/1 -> Logical3/1, Accumulator/3
  Logical3/1 -> Delay7/1
  Logical4/1 -> Logical3/2
  [new_mat] -> Logical4/1
  Constant6/1 -> Relational/2
  Constant5/1 -> Mux3/2
  Constant1/1 -> Mux3/3
  Accumulator/1 -> Relational/1
  Mux3/1 -> Accumulator/1
  [enable] -> Mux3/1

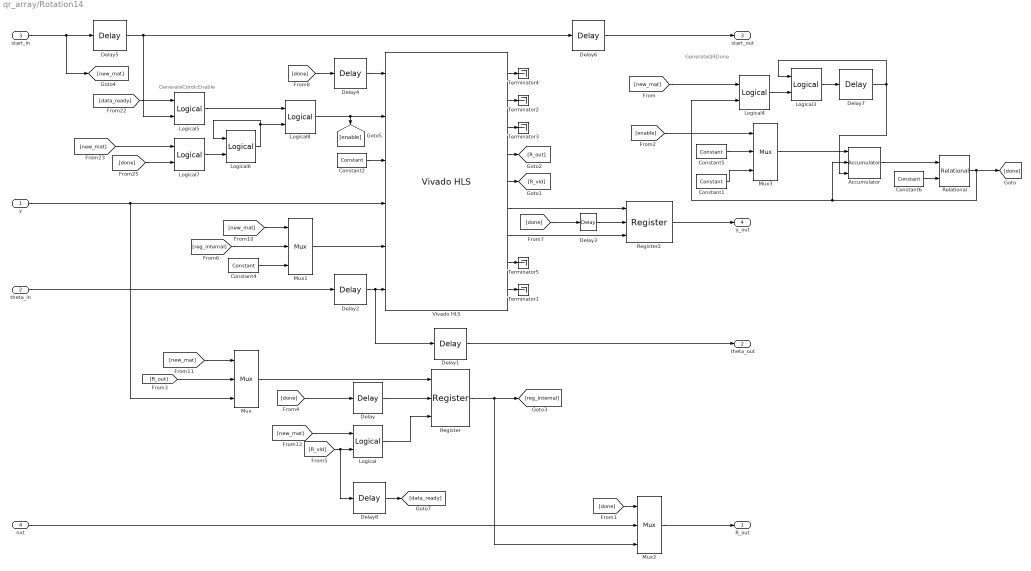
== system qr_array/Rotation14 ==
  note: GenerateQRDone
  note: GenerateCordicEnable
  y : Inport
  theta_in : Inport  Port=2
  start_in : Inport  Port=3
  nxt : Inport  Port=4
  Accumulator : xbsIndex_r4/Accumulator  operation=Add  n_bits=8  overflow=Wrap  scale=1  rst=on  hasbypass=off  infoeditControl=reset for floating point data type must be asserted for a minimum of 2 cycles  en=on  latency=1  msb_inp=100  msb=100  lsb=-100  use_behavioral_HDL=on  implementation=Fabric  dbl_ovrd=off  block_type=accum
  Constant1 : xbsIndex_r4/Constant  const=1  gui_display_data_type=Fixed-point  arith_type=Unsigned  n_bits=16  bin_pt=0  preci_type=Single  exp_width=8  frac_width=24  explicit_period=off  period=1  equ=P=C  opselect=C  inp2=PCIN>>17  opr=+  inp1=P  carry=CIN  dbl_ovrd=off  block_type=constant
  Constant2 : xbsIndex_r4/Constant  const=1  gui_display_data_type=Boolean  arith_type=Boolean  n_bits=16  bin_pt=14  preci_type=Single  exp_width=8  frac_width=24  explicit_period=off  period=1  equ=P=C  opselect=C  inp2=PCIN>>17  opr=+  inp1=P  carry=CIN  dbl_ovrd=off  block_type=constant
  Constant4 : xbsIndex_r4/Constant  const=0  gui_display_data_type=Fixed-point  arith_type=Signed (2's comp)  n_bits=16  bin_pt=13  preci_type=Single  exp_width=8  frac_width=24  explicit_period=off  period=1  equ=P=C  opselect=C  inp2=PCIN>>17  opr=+  inp1=P  carry=CIN  dbl_ovrd=off  block_type=constant
  Constant5 : xbsIndex_r4/Constant  const=0  gui_display_data_type=Fixed-point  arith_type=Unsigned  n_bits=16  bin_pt=0  preci_type=Single  exp_width=8  frac_width=24  explicit_period=off  period=1  equ=P=C  opselect=C  inp2=PCIN>>17  opr=+  inp1=P  carry=CIN  dbl_ovrd=off  block_type=constant
  Constant6 : xbsIndex_r4/Constant  const=2  gui_display_data_type=Fixed-point  arith_type=Unsigned  n_bits=16  bin_pt=0  preci_type=Single  exp_width=8  frac_width=24  explicit_period=off  period=1  equ=P=C  opselect=C  inp2=PCIN>>17  opr=+  inp1=P  carry=CIN  dbl_ovrd=off  block_type=constant
  Delay{,3,6..7} (4 alike) : xbsIndex_r4/Delay  rst=off  infoeditControl=Selection of Reset will increase slice count due to use of real FFs and instead of SRLs  en=off  latency=1  reg_retiming=off  dbl_ovrd=off  block_type=delay
  Delay1 : xbsIndex_r4/Delay  rst=off  infoeditControl=Selection of Reset will increase slice count due to use of real FFs and instead of SRLs  en=off  latency=41  reg_retiming=off  dbl_ovrd=off  block_type=delay
  Delay2 : xbsIndex_r4/Delay  rst=off  infoeditControl=Selection of Reset will increase slice count due to use of real FFs and instead of SRLs  en=off  latency=2  reg_retiming=off  dbl_ovrd=off  block_type=delay
  Delay4 : xbsIndex_r4/Delay  rst=off  infoeditControl=Selection of Reset will increase slice count due to use of real FFs and instead of SRLs  en=off  latency=4  reg_retiming=off  dbl_ovrd=off  block_type=delay
  Delay5 : xbsIndex_r4/Delay  rst=off  infoeditControl=Selection of Reset will increase slice count due to use of real FFs and instead of SRLs  en=off  latency=43  reg_retiming=off  dbl_ovrd=off  block_type=delay
  Delay8 : xbsIndex_r4/Delay  rst=off  infoeditControl=Selection of Reset will increase slice count due to use of real FFs and instead of SRLs  en=off  latency=2  reg_retiming=off  dbl_ovrd=off  block_type=delay
  Logical : xbsIndex_r4/Logical  logical_function=OR  inputs=2  en=off  latency=1  precision=Full  arith_type=Unsigned  n_bits=16  bin_pt=0  align_bp=on  dbl_ovrd=off  block_type=logical
  Logical3 : xbsIndex_r4/Logical  logical_function=XOR  inputs=2  en=off  latency=0  precision=Full  arith_type=Unsigned  n_bits=16  bin_pt=0  align_bp=on  dbl_ovrd=off  block_type=logical
  Logical4 : xbsIndex_r4/Logical  logical_function=OR  inputs=2  en=off  latency=1  precision=Full  arith_type=Unsigned  n_bits=16  bin_pt=0  align_bp=on  dbl_ovrd=off  block_type=logical
  Logical5 : xbsIndex_r4/Logical  logical_function=OR  inputs=2  en=off  latency=0  precision=Full  arith_type=Unsigned  n_bits=16  bin_pt=0  align_bp=on  dbl_ovrd=off  block_type=logical
  Logical6 : xbsIndex_r4/Logical  logical_function=XOR  inputs=2  en=off  latency=1  precision=Full  arith_type=Unsigned  n_bits=16  bin_pt=0  align_bp=on  dbl_ovrd=off  block_type=logical
  Logical7 : xbsIndex_r4/Logical  logical_function=OR  inputs=2  en=off  latency=1  precision=Full  arith_type=Unsigned  n_bits=16  bin_pt=0  align_bp=on  dbl_ovrd=off  block_type=logical
  Logical8 : xbsIndex_r4/Logical  logical_function=AND  inputs=2  en=off  latency=1  precision=Full  arith_type=Unsigned  n_bits=16  bin_pt=0  align_bp=on  dbl_ovrd=off  block_type=logical
  Mux{,1..3} (4 alike) : xbsIndex_r4/Mux  inputs=2  en=off  latency=1  precision=Full  arith_type=Unsigned  n_bits=16  bin_pt=14  quantization=Truncate  overflow=Wrap  dbl_ovrd=off  block_type=mux
  Register : xbsIndex_r4/Register  init=0  rst=on  en=on  dbl_ovrd=off  block_type=register
  Register2 : xbsIndex_r4/Register  init=0  rst=on  en=on  dbl_ovrd=off  block_type=register
  Relational : xbsIndex_r4/Relational  mode=a=b  op_type=Bool  en=off  latency=0  dbl_ovrd=off  block_type=relational
  Terminator{1..5} (5 alike) : Terminator
  Vivado HLS : xbsIndex_r4/Vivado HLS  anytable='C:/ELEC522/hellar/Project_4/cordic_revised/cordic_revised/solution1'  fast_sim=off  display_datatype=on  rate_propagation_method=Simulink system period  model_file_path=''  latency=1  block_type=hls
      settings: infoedit=This block allows including C,C++ and SystemC source files in System Generator for DSP designs.
  R_out : Outport
  theta_out : Outport  Port=2
  start_out : Outport  Port=3
  y_out : Outport  Port=4
  wires:
  [done] -> Delay3/1
  Delay8/1 -> [data_ready]
  [R_vld] -> Delay8/1, Logical/2
  [done] -> Mux2/1
  [new_mat] -> Mux/1
  [done] -> Delay4/1
  [new_mat] -> Mux1/1
  [reg_internal] -> Mux1/2
  Delay4/1 -> Vivado HLS/1
  Logical/1 -> Register/3
  [done] -> Delay/1
  [new_mat] -> Logical/1
  theta_in/1 -> Delay2/1
  Register/1 -> Mux2/3, [reg_internal]
  Delay6/1 -> start_out/1
  Mux/1 -> Register/1
  Vivado HLS/3 -> Terminator3/1
  Vivado HLS/5 -> [R_vld]
  [R_out] -> Mux/2
  Delay/1 -> Register/2
  y/1 -> Vivado HLS/4, Mux/3
  Vivado HLS/1 -> Terminator4/1
  Vivado HLS/4 -> [R_out]
  Mux2/1 -> R_out/1
  Constant4/1 -> Mux1/3
  start_in/1 -> [new_mat], Delay5/1
  nxt/1 -> Mux2/2
  Vivado HLS/2 -> Terminator2/1
  Constant2/1 -> Vivado HLS/3
  Logical8/1 -> Vivado HLS/2, [enable]
  Relational/1 -> Logical4/2, Accumulator/2, [done]
  Vivado HLS/8 -> Terminator5/1
  Vivado HLS/9 -> Terminator1/1
  Vivado HLS/6 -> Register2/1
  Vivado HLS/7 -> Register2/3
  Delay1/1 -> theta_out/1
  Delay2/1 -> Delay1/1, Vivado HLS/6
  Mux1/1 -> Vivado HLS/5
  Delay3/1 -> Register2/2
  Register2/1 -> y_out/1
  Logical5/1 -> Logical8/1
  Logical7/1 -> Logical6/2
  Logical6/1 -> Logical6/1, Logical8/2
  [done] -> Logical7/2
  [new_mat] -> Logical7/1
  [data_ready] -> Logical5/1
  Delay5/1 -> Delay6/1, Logical5/2
  Delay7/1 -> Logical3/1, Accumulator/3
  Logical3/1 -> Delay7/1
  Logical4/1 -> Logical3/2
  [new_mat] -> Logical4/1
  Constant6/1 -> Relational/2
  Constant5/1 -> Mux3/2
  Constant1/1 -> Mux3/3
  Accumulator/1 -> Relational/1
  Mux3/1 -> Accumulator/1
  [enable] -> Mux3/1

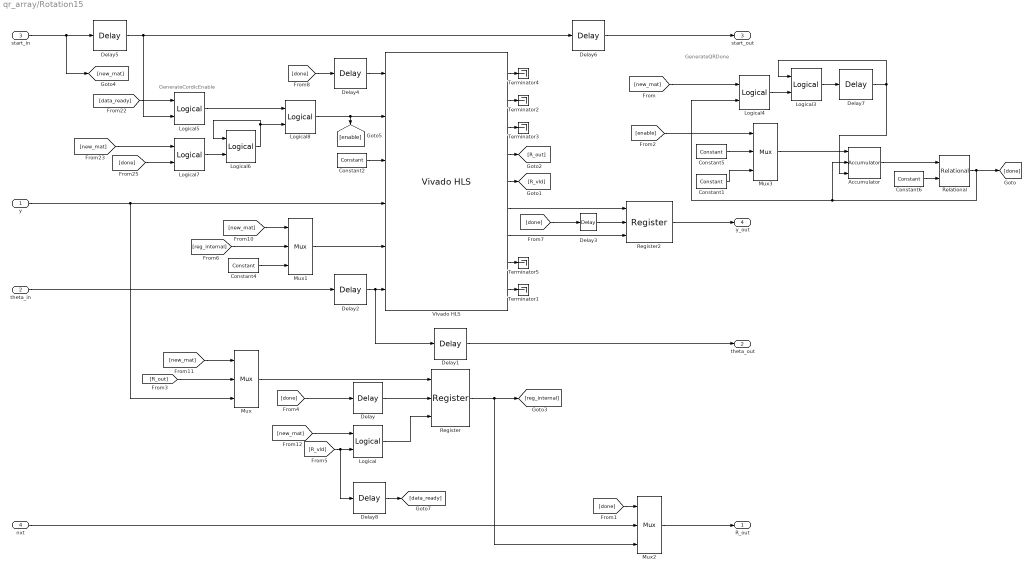
== system qr_array/Rotation15 ==
  note: GenerateQRDone
  note: GenerateCordicEnable
  y : Inport
  theta_in : Inport  Port=2
  start_in : Inport  Port=3
  nxt : Inport  Port=4
  Accumulator : xbsIndex_r4/Accumulator  operation=Add  n_bits=8  overflow=Wrap  scale=1  rst=on  hasbypass=off  infoeditControl=reset for floating point data type must be asserted for a minimum of 2 cycles  en=on  latency=1  msb_inp=100  msb=100  lsb=-100  use_behavioral_HDL=on  implementation=Fabric  dbl_ovrd=off  block_type=accum
  Constant1 : xbsIndex_r4/Constant  const=1  gui_display_data_type=Fixed-point  arith_type=Unsigned  n_bits=16  bin_pt=0  preci_type=Single  exp_width=8  frac_width=24  explicit_period=off  period=1  equ=P=C  opselect=C  inp2=PCIN>>17  opr=+  inp1=P  carry=CIN  dbl_ovrd=off  block_type=constant
  Constant2 : xbsIndex_r4/Constant  const=1  gui_display_data_type=Boolean  arith_type=Boolean  n_bits=16  bin_pt=14  preci_type=Single  exp_width=8  frac_width=24  explicit_period=off  period=1  equ=P=C  opselect=C  inp2=PCIN>>17  opr=+  inp1=P  carry=CIN  dbl_ovrd=off  block_type=constant
  Constant4 : xbsIndex_r4/Constant  const=0  gui_display_data_type=Fixed-point  arith_type=Signed (2's comp)  n_bits=16  bin_pt=13  preci_type=Single  exp_width=8  frac_width=24  explicit_period=off  period=1  equ=P=C  opselect=C  inp2=PCIN>>17  opr=+  inp1=P  carry=CIN  dbl_ovrd=off  block_type=constant
  Constant5 : xbsIndex_r4/Constant  const=0  gui_display_data_type=Fixed-point  arith_type=Unsigned  n_bits=16  bin_pt=0  preci_type=Single  exp_width=8  frac_width=24  explicit_period=off  period=1  equ=P=C  opselect=C  inp2=PCIN>>17  opr=+  inp1=P  carry=CIN  dbl_ovrd=off  block_type=constant
  Constant6 : xbsIndex_r4/Constant  const=2  gui_display_data_type=Fixed-point  arith_type=Unsigned  n_bits=16  bin_pt=0  preci_type=Single  exp_width=8  frac_width=24  explicit_period=off  period=1  equ=P=C  opselect=C  inp2=PCIN>>17  opr=+  inp1=P  carry=CIN  dbl_ovrd=off  block_type=constant
  Delay{,3,6..7} (4 alike) : xbsIndex_r4/Delay  rst=off  infoeditControl=Selection of Reset will increase slice count due to use of real FFs and instead of SRLs  en=off  latency=1  reg_retiming=off  dbl_ovrd=off  block_type=delay
  Delay1 : xbsIndex_r4/Delay  rst=off  infoeditControl=Selection of Reset will increase slice count due to use of real FFs and instead of SRLs  en=off  latency=41  reg_retiming=off  dbl_ovrd=off  block_type=delay
  Delay2 : xbsIndex_r4/Delay  rst=off  infoeditControl=Selection of Reset will increase slice count due to use of real FFs and instead of SRLs  en=off  latency=2  reg_retiming=off  dbl_ovrd=off  block_type=delay
  Delay4 : xbsIndex_r4/Delay  rst=off  infoeditControl=Selection of Reset will increase slice count due to use of real FFs and instead of SRLs  en=off  latency=4  reg_retiming=off  dbl_ovrd=off  block_type=delay
  Delay5 : xbsIndex_r4/Delay  rst=off  infoeditControl=Selection of Reset will increase slice count due to use of real FFs and instead of SRLs  en=off  latency=43  reg_retiming=off  dbl_ovrd=off  block_type=delay
  Delay8 : xbsIndex_r4/Delay  rst=off  infoeditControl=Selection of Reset will increase slice count due to use of real FFs and instead of SRLs  en=off  latency=2  reg_retiming=off  dbl_ovrd=off  block_type=delay
  Logical : xbsIndex_r4/Logical  logical_function=OR  inputs=2  en=off  latency=1  precision=Full  arith_type=Unsigned  n_bits=16  bin_pt=0  align_bp=on  dbl_ovrd=off  block_type=logical
  Logical3 : xbsIndex_r4/Logical  logical_function=XOR  inputs=2  en=off  latency=0  precision=Full  arith_type=Unsigned  n_bits=16  bin_pt=0  align_bp=on  dbl_ovrd=off  block_type=logical
  Logical4 : xbsIndex_r4/Logical  logical_function=OR  inputs=2  en=off  latency=1  precision=Full  arith_type=Unsigned  n_bits=16  bin_pt=0  align_bp=on  dbl_ovrd=off  block_type=logical
  Logical5 : xbsIndex_r4/Logical  logical_function=OR  inputs=2  en=off  latency=0  precision=Full  arith_type=Unsigned  n_bits=16  bin_pt=0  align_bp=on  dbl_ovrd=off  block_type=logical
  Logical6 : xbsIndex_r4/Logical  logical_function=XOR  inputs=2  en=off  latency=1  precision=Full  arith_type=Unsigned  n_bits=16  bin_pt=0  align_bp=on  dbl_ovrd=off  block_type=logical
  Logical7 : xbsIndex_r4/Logical  logical_function=OR  inputs=2  en=off  latency=1  precision=Full  arith_type=Unsigned  n_bits=16  bin_pt=0  align_bp=on  dbl_ovrd=off  block_type=logical
  Logical8 : xbsIndex_r4/Logical  logical_function=AND  inputs=2  en=off  latency=1  precision=Full  arith_type=Unsigned  n_bits=16  bin_pt=0  align_bp=on  dbl_ovrd=off  block_type=logical
  Mux{,1..3} (4 alike) : xbsIndex_r4/Mux  inputs=2  en=off  latency=1  precision=Full  arith_type=Unsigned  n_bits=16  bin_pt=14  quantization=Truncate  overflow=Wrap  dbl_ovrd=off  block_type=mux
  Register : xbsIndex_r4/Register  init=0  rst=on  en=on  dbl_ovrd=off  block_type=register
  Register2 : xbsIndex_r4/Register  init=0  rst=on  en=on  dbl_ovrd=off  block_type=register
  Relational : xbsIndex_r4/Relational  mode=a=b  op_type=Bool  en=off  latency=0  dbl_ovrd=off  block_type=relational
  Terminator{1..5} (5 alike) : Terminator
  Vivado HLS : xbsIndex_r4/Vivado HLS  anytable='C:/ELEC522/hellar/Project_4/cordic_revised/cordic_revised/solution1'  fast_sim=off  display_datatype=on  rate_propagation_method=Simulink system period  model_file_path=''  latency=1  block_type=hls
      settings: infoedit=This block allows including C,C++ and SystemC source files in System Generator for DSP designs.
  R_out : Outport
  theta_out : Outport  Port=2
  start_out : Outport  Port=3
  y_out : Outport  Port=4
  wires:
  [done] -> Delay3/1
  Delay8/1 -> [data_ready]
  [R_vld] -> Delay8/1, Logical/2
  [done] -> Mux2/1
  [new_mat] -> Mux/1
  [done] -> Delay4/1
  [new_mat] -> Mux1/1
  [reg_internal] -> Mux1/2
  Delay4/1 -> Vivado HLS/1
  Logical/1 -> Register/3
  [done] -> Delay/1
  [new_mat] -> Logical/1
  theta_in/1 -> Delay2/1
  Register/1 -> Mux2/3, [reg_internal]
  Delay6/1 -> start_out/1
  Mux/1 -> Register/1
  Vivado HLS/3 -> Terminator3/1
  Vivado HLS/5 -> [R_vld]
  [R_out] -> Mux/2
  Delay/1 -> Register/2
  y/1 -> Vivado HLS/4, Mux/3
  Vivado HLS/1 -> Terminator4/1
  Vivado HLS/4 -> [R_out]
  Mux2/1 -> R_out/1
  Constant4/1 -> Mux1/3
  start_in/1 -> [new_mat], Delay5/1
  nxt/1 -> Mux2/2
  Vivado HLS/2 -> Terminator2/1
  Constant2/1 -> Vivado HLS/3
  Logical8/1 -> Vivado HLS/2, [enable]
  Relational/1 -> Logical4/2, Accumulator/2, [done]
  Vivado HLS/8 -> Terminator5/1
  Vivado HLS/9 -> Terminator1/1
  Vivado HLS/6 -> Register2/1
  Vivado HLS/7 -> Register2/3
  Delay1/1 -> theta_out/1
  Delay2/1 -> Delay1/1, Vivado HLS/6
  Mux1/1 -> Vivado HLS/5
  Delay3/1 -> Register2/2
  Register2/1 -> y_out/1
  Logical5/1 -> Logical8/1
  Logical7/1 -> Logical6/2
  Logical6/1 -> Logical6/1, Logical8/2
  [done] -> Logical7/2
  [new_mat] -> Logical7/1
  [data_ready] -> Logical5/1
  Delay5/1 -> Delay6/1, Logical5/2
  Delay7/1 -> Logical3/1, Accumulator/3
  Logical3/1 -> Delay7/1
  Logical4/1 -> Logical3/2
  [new_mat] -> Logical4/1
  Constant6/1 -> Relational/2
  Constant5/1 -> Mux3/2
  Constant1/1 -> Mux3/3
  Accumulator/1 -> Relational/1
  Mux3/1 -> Accumulator/1
  [enable] -> Mux3/1
